simulink library "dsda_lib"  (R2021b)
settings: Solver=VariableStepAuto  StartTime=0.0  StopTime=10.0  RelTol=1e-3
libraries: $bdroot x1, simulink x1
settings Model: Creator=schwammw  LastModifiedBy=schwammw

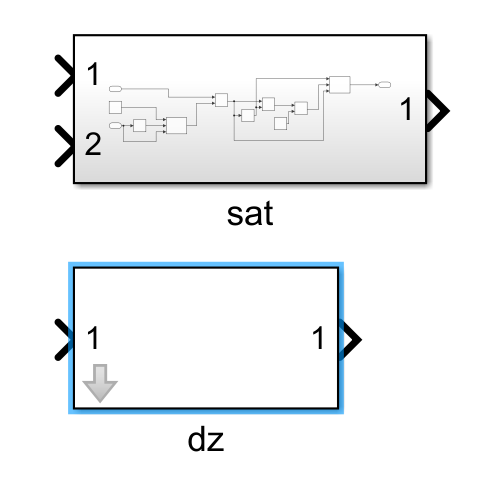
[thumbnail: Simulink's stored preview of the top-level diagram]
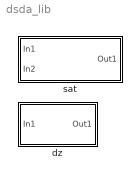
== system dsda_lib ==
  dz : Subsystem  mask{ulim=1}
      mask prompts: ulim "Karina"
  sat : Subsystem

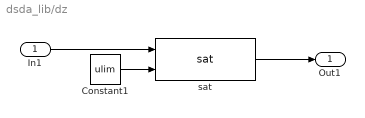
== system dsda_lib/dz ==
  In1 : Inport
  Constant1 : Constant  Value=ulim  SampleTime=-1
  sat : $bdroot/sat  SystemSampleTime=-1  VariantActivationTime=update diagram  Latency=0  AutoFrameSizeCalculation=off
  Out1 : Outport
  wires:
  In1/1 -> sat/1
  sat/1 -> Out1/1
  Constant1/1 -> sat/2

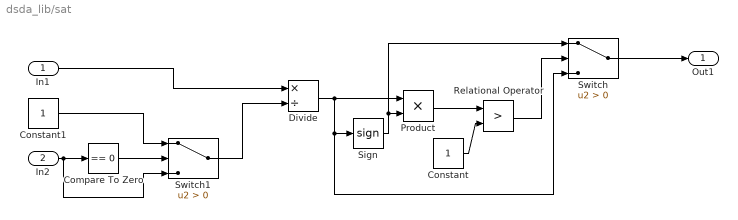
== system dsda_lib/sat ==
  In1 : Inport
  In2 : Inport  Port=2
  Compare To Zero : simulink/Logic and Bit Operations/Compare To Zero  relop===  OutDataTypeStr=boolean
  Constant : Constant  SampleTime=-1
  Constant1 : Constant  SampleTime=-1
  Divide : Product  Inputs=*/
  Product : Product
  Relational Operator : RelationalOperator  Operator=>  OutDataTypeStr=boolean  RndMeth=Simplest
  Sign : Signum
  Switch : Switch  Criteria=u2 > Threshold
  Switch1 : Switch  Criteria=u2 > Threshold
  Out1 : Outport
  wires:
  Compare To Zero/1 -> Switch1/2
  Constant1/1 -> Switch1/1
  In2/1 -> Compare To Zero/1, Switch1/3
  Switch/1 -> Out1/1
  Relational Operator/1 -> Switch/2
  Product/1 -> Relational Operator/1
  Sign/1 -> Product/2, Switch/1
  Divide/1 -> Product/1, Switch/3, Sign/1
  Switch1/1 -> Divide/2
  In1/1 -> Divide/1
  Constant/1 -> Relational Operator/2
